simulink model "deterministicAttitude"  (R2023b)
settings: Solver=VariableStepAuto  StartTime=0.0  StopTime=Tfinal  RelTol=1e-3
libraries: matrix_library x1
settings Model: Creator=kristopherriordan  LastModifiedBy=kristopherriordan

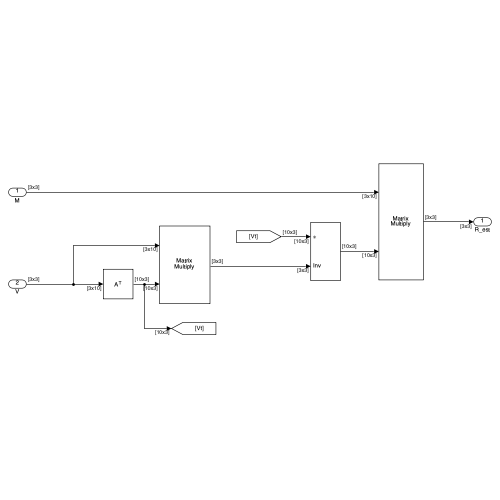
[thumbnail: Simulink's stored preview of the top-level diagram]
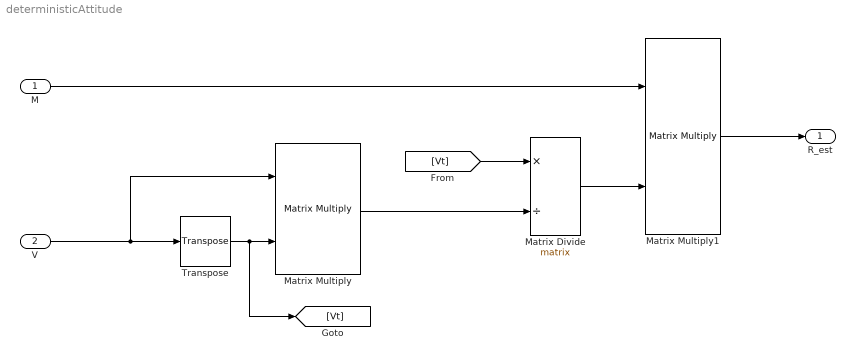
== system deterministicAttitude ==
  M : Inport  PortDimensions=[3 3]
  V : Inport  Port=2  PortDimensions=[3 3]
  Matrix Divide : Product  Inputs=*/  Multiplication=Matrix(*)
  Matrix Multiply : Product  Inputs=**  Multiplication=Matrix(*)
  Matrix Multiply1 : Product  Inputs=**  Multiplication=Matrix(*)
  Transpose : matrix_library/Transpose
  R_est : Outport  PortDimensions=[3 3]
  wires:
  M/1 -> Matrix Multiply1/1
  V/1 -> Matrix Multiply/1, Transpose/1
  Transpose/1 -> [Vt], Matrix Multiply/2
  [Vt] -> Matrix Divide/1
  Matrix Multiply/1 -> Matrix Divide/2
  Matrix Divide/1 -> Matrix Multiply1/2
  Matrix Multiply1/1 -> R_est/1
